simulink model "AgrivoltaicPlatformBasic5_28"  (R2023b)
settings: Solver=VariableStepAuto  StartTime=0.0  StopTime=Tsim  RelTol=1e-3
undefined symbols (not defined in the file or in its folder): Boostparams, Buckparams, Ion, Lithium, PVparams
libraries: fl_lib x18, ee_lib x8, spsSeriesRLCBranchLib x6, nesl_utility x6, spsDiodeLib x2, spsMosfetLib x2, spsPVArrayLib x2, spsVoltageMeasurementLib x2, spsBatteryLib x1, spsCurrentVoltageSimscapeInterfaceLib x1, spsGroundLib x1, sps_lib x1
settings Model: Creator=akoer  LastModifiedBy=akoer
settings DebuggingCC: SignalInfNanChecking=error

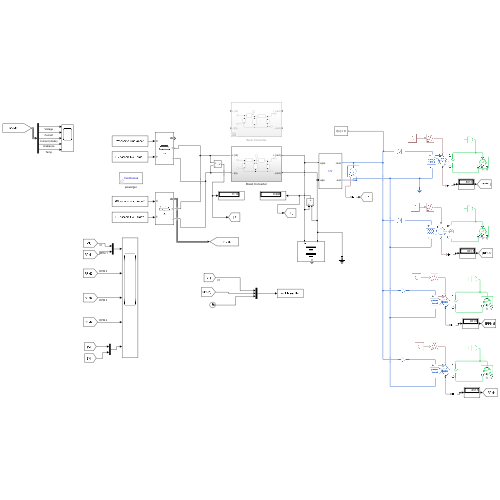
[thumbnail: Simulink's stored preview of the top-level diagram]
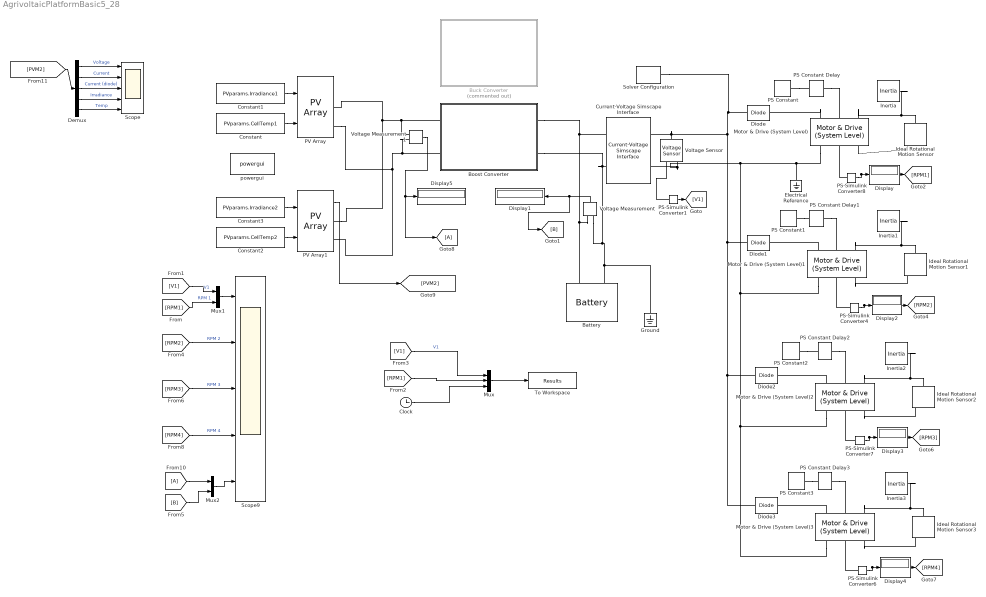
== system AgrivoltaicPlatformBasic5_28 ==
  Battery : spsBatteryLib/Battery  BatType=Lithium-Ion  ShowTempParam=off  ThermalPreset=no  ShowAgeParam=off  NomV=7.2  NomQ=20  SOC=20  Batt_Tr=30  PresetModel=on  MaxQ=20  MinV=5.4  FullV=8.3807  Dis_rate=8.6957  R=0.0036  Normal_OP=18.087  expZone="[7.7788     0.98261]"  current=[6.5 13 32.5]  Units=Time  Tci=20  NomT=20  T2=-30  MaxQ2=4.8  FullV2=7.1  Normal_OP2=5.655  expZone2="[6.58           1]"  Rca=0.6  ti=2000  Dp=0  Neq0=0  Tsim=1e6  Ta1=25  Qeol=5.4*0.9  Reol=0.013333*1.2  Char_age=[2.3478, 3]  Dis_age=[2.3478, 10]  N1=1500  N2=10500  N3=1000  N4=1400  Ta2=45  N5=950
  Boost Converter : Subsystem
  Buck Converter : Subsystem  Commented=on
  Clock : Clock
  Constant : Constant  Value=PVparams.CellTemp1
  Constant1 : Constant  Value=PVparams.Irradiance1
  Constant2 : Constant  Value=PVparams.CellTemp2
  Constant3 : Constant  Value=PVparams.Irradiance2
  Current-Voltage Simscape Interface : spsCurrentVoltageSimscapeInterfaceLib/Current-Voltage Simscape Interface  DFT=on  FMode=Low pass filter (continuous)  T=1e-6  Ts=50e-6  i0=0  v0=0  Sd=Specialized Power Systems side  Measurements=off
      settings: LibrarySourceBlock=|
      | sps_lib/Utilities/Current-Voltage
      | Simscape Interface
  Demux : Demux  Outputs=5
  Diode{,1..3} (4 alike) : ee_lib/Semiconductors & Converters/Diode  ModelType=ee.enum.diode.modelType.pwl  TableType=ee.enum.diode.tableType.IfMat  IfMat=[.07, .12, .19, 1.75, 4.24, 7.32, 11.2; .16, .3, .72, 2.14, 5.02, 8.35, 13.12] A  VfMat=[.9, 1.15, 1.25, 1.5, 1.75, 2.17, 2.6, 2.85; .58, .68, .75, 1.1, 1.38, 1.77, 2.27, 2.7] V  TjVec=[25, 125] degC  VfVec=[.5, .7, .9, 1.3, 1.7, 2.1, 2.5] V  IfVec=[.1, .2, .5, 1, 2, 4, 7, 10] A  Vf=0.6 V  Ron=0.3 Ohm  Goff=1e-8 S  prmExp=ee.enum.diode.expParam.useTwo  I12=[.0137, .545] A  V12=[.6, .7] V  RS=0 Ohm  Tmeas=25 degC  IS=1e-12 A  ec=1  I1=0.0137 A  V1=0.6 V  N_series=1  N_parallel=1  ZenerEnable=false  Rz=0.3 Ohm  BV=inf V  C_param=ee.enum.diode.capParam.fixed  CJ=0 pF  CJ0=5 pF  Vvec=[.1, 10, 100] V  Cvec=[3.5, 1, .4] pF  VJ=1 V  Mgrad=0.5  FC=0.5  Q_param=ee.enum.diode.recoveryParam.off  iRM=-7.15 A  iF=4 A  didt=-750 A/us  trr_factor=3  trr=115 ns  Qrr=150 nA*s  Vr=-600 V  Ls=150 nH  Erec=0.03 J  TT=50 ns  tau=100 ns  T_param=ee.enum.diode.temperatureParam.off  Tdevice=25 degC  I1_T2=0.245 A  V1_T2=0.5 V  IS_T2=1.25e-7 A  Tmeas2=125 degC  XTI_param=ee.enum.diode.xtiParam.pn  XTI=3  EG_param=ee.enum.diode.egapParam.material_si  EG=1.11 eV  dBVdT=0 V/K  enable_faults=simscape.enum.onoff.off  fault_action=simscape.enum.assert.action.none  fault_types=ee.enum.diode.faults.open  tau_fault=1e-3 s  IfMat_faulted=[.07, .12, .19, 1.75, 4.24, 7.32, 11.2; .16, .3, .72, 2.14, 4.02, 6.35, 9.12] A  VfMat_faulted=[.9, 1.15, 1.25, 1.5, 1.75, 2.17, 2.6, 2.85; .58, .68, .75, 1.1, 1.38, 1.77, 2.27, 2.7] V  VfVec_faulted=[.5, .7, .9, 1.3, 1.7, 2.1, 2.5] V  IfVec_faulted=[.1, .2, .5, 1, 2, 4, 7, 10] A  Ropen_faulted=1000 Ohm  Gshort_faulted=1000 1/Ohm  Vf_faulted=0.6 V  Ron_faulted=0.3 Ohm  Goff_faulted=1e-8 S  I12_faulted=[.0137, .545] A  V12_faulted=[.6, .7] V  IS_faulted=1e-12 A  ec_faulted=1  I1_faulted=0.0137 A  V1_faulted=0.6 V  RS_faulted=0 Ohm  Rz_faulted=0.3 Ohm  BV_faulted=inf V  Cscale_faulted=100  fault_trigger=ee.enum.faults.faultTrigger.temporal  t_fault=inf s  max_permissible_voltage=inf V  n_fail_on_voltage=1  max_permissible_current=inf A  t_fail_on_current=1 s  max_permissible_dVdt=inf V/s  enable_fault_input=simscape.enum.onoff.off  i_specify=off  i_priority=None  i=0 A  i_nominal_specify=off  i_nominal_unit=A  i_nominal_value=1  v_specify=off  v_priority=None  v=0 V  v_nominal_specify=off  v_nominal_unit=V  v_nominal_value=1  v_capacitor_specify=off  v_capacitor_priority=None  v_capacitor=0 V  v_capacitor_nominal_specify=off  v_capacitor_nominal_unit=V  v_capacitor_nominal_value=1  faulted_specify=off  faulted_priority=None  faulted=0  faulted_nominal_specify=off  faulted_nominal_unit=1  faulted_nominal_value=1  i_diode_specify=off  i_diode_priority=None  i_diode=0 A  i_diode_nominal_specify=off  i_diode_nominal_unit=A  i_diode_nominal_value=1  v_diode_specify=off  v_diode_priority=None  v_diode=0 V  v_diode_nominal_specify=off  v_diode_nominal_unit=V  v_diode_nominal_value=1  i_capacitor_specify=off  i_capacitor_priority=None  i_capacitor=0 A  i_capacitor_nominal_specify=off  i_capacitor_nominal_unit=A  i_capacitor_nominal_value=1  power_dissipated_specify=off  power_dissipated_priority=None  power_dissipated=0 W  power_dissipated_nominal_specify=off  power_dissipated_nominal_unit=W  power_dissipated_nominal_value=1  fidelity_level=ee.enum.diode.fidelity.includeChargeDyn  rec_loss_model=ee.enum.diode.reverseRecoveryModel.fixed  ErecVal=0 J  scaleWithIandV=true  ErecMat=zeros(2, 3) J  TjrecVec=[298.15, 398.15] K  IfrecVec=[.1, 1, 10] A  IrecVal=10 A  VrecVal=10 V  tFilter=1 / 1000 / 100 s  max_permissible_temperature=inf K  t_fail_on_temperature=1 s  thermal_network_parameterization=ee.enum.thermalNetworkTopology.junctionCase  Rth=[0, 10] K/W  Rth_Cauer=[1, 3, 10] K/W  Rth_Foster=[4, 6] K/W  thermal_mass_parameterization=ee.enum.thermalNetwork.timeconstant  thermal_mass=[0, 1] J/K  thermal_mass_Cauer=[.1, .3, 1] J/K  thermal_mass_Foster=[1.5, 3] J/K  thermal_time_constant=[0, 10] s  thermal_time_constant_Cauer=[1, 3, 10] s  thermal_time_constant_Foster=[6, 18] s  thermal_mass_initial_temperatures=[25, 25] degC  thermal_mass_initial_temperatures_Cauer=[25, 25, 25] degC  junction_thermal_mass=0.01 J/K  Tvec_initial_Foster=[25, 25, 25, 25] degC  no_thermal_network=0  junction_temperature_specify=off  junction_temperature_priority=None  junction_temperature=25 degC  junction_temperature_nominal_specify=off  junction_temperature_nominal_unit=degC  junction_temperature_nominal_value=1
  Display{,1..5} (6 alike) : Display
  Electrical Reference : fl_lib/Electrical/Electrical Elements/Electrical Reference
  From10 : From
  Goto8 : Goto
  Ground : spsGroundLib/Ground  LConnTagsString=a
  Ideal Rotational Motion Sensor{,1..3} (4 alike) : fl_lib/Mechanical/Mechanical Sensors/Ideal Rotational Motion Sensor  reference=foundation.enum.MeasurementReference.difference  acceleration_port=false  velocity_port=true  position_port=true  wrap_angle=false  offset=0 rad
  Inertia{,1..3} (4 alike) : fl_lib/Mechanical/Rotational Elements/Inertia  inertia=params.Inertia kg*m^2  num_ports=foundation.enum.numPorts2.one  w_specify=off  w_priority=High  w=0 rad/s  w_nominal_specify=off  w_nominal_unit=rad/s  w_nominal_value=1  t_specify=off  t_priority=None  t=0 N*m  t_nominal_specify=off  t_nominal_unit=N*m  t_nominal_value=1
  Motor & Drive (System Level){,1..3} (4 alike) : ee_lib/Electromechanical/Motor & Drive (System Level)  torque_speed_param=ee.enum.electromech.envelope.tabulated2D  overtorque_param=ee.enum.electromech.overtorque.no  T_t=[.09, .08, .07, 0] N*m  T_t_intermittent=[.36, .32, .28, 0] N*m  T_t_2D=[.09, .09, .09; .08, .08, .08; .07, .07, .07; 0, 0, 0] N*m  T_t_intermittent_2D=[.36, .36, .36; .32, .32, .32; .28, .28, .28; 0, 0, 0] N*m  w_t=[0, 3750, 7500, 8000] rpm  vdc_t=[6, 12, 24] V  torque_max=0.1 N*m  power_max=30 W  torque_max_intermittent=0.4 N*m  power_max_intermittent=120 W  time_overtorque=30 s  time_recover=60 s  Tc=0.02 s  EnableSwitch=false  losses_param=1  eff=100  w_eff=3750 rpm  T_eff=0.08 N*m  Piron=0 W  Pbase=0 W  w_eff_vec=[-8000, -4000, 0, 4000, 8000] rpm  T_eff_vec=[0, .03, .06, .09] N*m  v_eff_vec=[100, 250, 400] V  losses_mat=[1.49, 1.67, 2.21, 3.1; .42, .69, 1.14, 2.03; .06, .24, .78, 1.68; .42, .69, 1.14, 2.03; 1.49, 1.67, 2.21, 3.1] W  efficiency_mat=[95, 95, 95, 95; 95, 95, 95, 95; 95, 95, 95, 95; 95, 95, 95, 95; 95, 95, 95, 95]  losses_mat_3D=ones(5, 4, 3) W  efficiency_mat_3D=95 * ones(5, 4, 3)  Res=0 Ohm  enable_fault=simscape.enum.onoff.off  fault_condition=1  fault_threshold=0.5  J=5e-5 kg*m^2  lam=1e-5 N*m*s/rad  speed0=0 rpm  faulted_specify=off  faulted_priority=None  faulted=0  faulted_nominal_specify=off  faulted_nominal_unit=1  faulted_nominal_value=1  isSwitchedOff_specify=off  isSwitchedOff_priority=None  isSwitchedOff=0  isSwitchedOff_nominal_specify=off  isSwitchedOff_nominal_unit=1  isSwitchedOff_nominal_value=1  torqueLimitContinuous_specify=off  torqueLimitContinuous_priority=None  torqueLimitContinuous=0 N*m  torqueLimitContinuous_nominal_specify=off  torqueLimitContinuous_nominal_unit=N*m  torqueLimitContinuous_nominal_value=1  alpha=3.93e-3 1/K  Tmeas=25 degC  Tmeas2=125 degC  losses_mat_T2=[1.49, 1.74, 2.49, 3.74; .42, .67, 1.42, 2.67; .06, .31, 1.06, 2.31; .42, .67, 1.42, 2.67; 1.49, 1.74, 2.49, 3.74] W  efficiency_mat_T2=[95, 95, 95, 95; 95, 95, 95, 95; 95, 95, 95, 95; 95, 95, 95, 95; 95, 95, 95, 95]  losses_mat_3D_T2=ones(5, 4, 3) W  efficiency_mat_3D_T2=95 * ones(5, 4, 3)  thermal_mass=100 J/K  initial_temperature=25 degC
  Mux : Mux  Inputs=3
  Mux1 : Mux  Inputs=2
  Mux2 : Mux  Inputs=2
  PS Constant : fl_lib/Physical Signals/Sources/PS Constant  constant=params.Torque1 N*m
  PS Constant Delay{,1..3} (4 alike) : fl_lib/Physical Signals/Delays/PS Constant Delay  InputHistory=0.0 N*m  DelayTime=1.0 s
      settings: InternalSimscapePortConfiguration="{\"Bottom\":[],\"Left\":[{\"id\":\"U\",\"label\":\"U\",\"type\":\"input\"}],\"Right\":[{\"id\":\"Y\",\"label\":\"Y\",\"type\":\"output\"}],\"Top\":[]}"
  PS Constant1 : fl_lib/Physical Signals/Sources/PS Constant  constant=params.Torque2 N*m
  PS Constant2 : fl_lib/Physical Signals/Sources/PS Constant  constant=params.Torque3 N*m
  PS Constant3 : fl_lib/Physical Signals/Sources/PS Constant  constant=params.Torque4 N*m
  PS-Simulink Converter{1,4,6..8} (5 alike) : nesl_utility/PS-Simulink Converter  PhysicalDomain=network_engine_domain  SubClassName=ps_output  LeftPortType=input  RightPortType=output  PseudoPeriodic=off  Frequencies=[]  VectorFormat=inherit  Unit=inherit  AffineConversion=off
  PV Array : spsPVArrayLib/PV Array  Npar=PVparams.Parallel1  Nser=PVparams.Series1  PlotType=array @ 1000 W/m2 & specified temperatures  S_vec="[ 1000  500  100 ]"  Temp_C_vec="[ 45 25  ]"  ModuleName=American Solar Wholesale ASW-185M  PlotWhenSelected=off  Pm=185.13  Ncell=72  Voc=44.6  Isc=5.37  Vm=37.4  Im=4.95  beta_Voc_pc=-0.38595  alpha_Isc_pc=0.043594  beta_Voc=-0.17213  alpha_Isc=0.002341  IL=5.3768  I0=4.1873e-10  nI=1.0375  Rsh=226.7768  Rs=0.28792  RobustModel=off  RobustCellTemperature=313.3991  BAL=on  Tc=1e-6  Tfilter=5e-5
  PV Array1 : spsPVArrayLib/PV Array  Npar=PVparams.Parallel2  Nser=PVparams.Series2  PlotType=array @ 1000 W/m2 & specified temperatures  S_vec="[ 1000  500  100 ]"  Temp_C_vec="[ 45 25  ]"  ModuleName=American Solar Wholesale ASW-185M  PlotWhenSelected=off  Pm=185.13  Ncell=72  Voc=44.6  Isc=5.37  Vm=37.4  Im=4.95  beta_Voc_pc=-0.38595  alpha_Isc_pc=0.043594  beta_Voc=-0.17213  alpha_Isc=0.002341  IL=5.3768  I0=4.1873e-10  nI=1.0375  Rsh=226.7768  Rs=0.28792  RobustModel=off  RobustCellTemperature=313.3991  BAL=on  Tc=1e-6  Tfilter=5e-5
  Scope : Scope  NumInputPorts=5
  Scope9 : Scope  NumInputPorts=5
  Solver Configuration : nesl_utility/Solver Configuration  PhysicalDomain=network_engine_domain  SubClassName=solver  LeftPortType=input  RightPortType=generic  Tones=[]  Harmonics=[]  SimulateNoise=off  Profile=off  UseLocalSampling=off  EnableSwitchedLinearOptims=on  FrequencyDomain=off  UseCCode=off  RelTol=0.001  AbsTol=0.001  MinStep=1e-09  ToWorkspace=off  RevertToSquareIcSolve=off  NumHomotopyIterations=100  PhasorMode=off  PhasorModeNumHarmonics=1  ConsistencySolver=NEWTON_XTOL_AFTER_FTOL  IndexReductionMethod=DerivativeReplacement  DoDC=off  ResidualTolerance=1e-09  ConsistencyTolSource=GLOBAL  ConsistencyAbsTol=0.001  ConsistencyRelTol=0.001  ConsistencyTolFactor=0.001  UseLocalSolver=off  LocalSolverChoice=NE_BACKWARD_EULER_ADVANCER  ResolveIndetEquations=on  FunctionEvalNumThread=1  LocalSolverSampleTime=0.001  DoFixedCost=off  MaxNonlinIter=3  MaxModeIter=2  ComputeImpulses=off  ImpulseIterations=2  LinearAlgebra=auto  LinearAlgebraNumThread=0  EquationFormulation=NE_TIME_EF  DelaysMemoryBudget=1024  AutomaticFiltering=on  FilteringTimeConstant=0.001  PartitionStorageMethod=AS_NEEDED  PartitionMemoryBudget=1024  PartitionMethod=ROBUST  MultibodyUseLocalSolver=off  MultibodyLocalSolverChoice=ODE1  MultibodyLocalSolverSampleTime=0.001
  To Workspace : ToWorkspace  VariableName=Results  SampleTime=-1
  Voltage Measurement : spsVoltageMeasurementLib/Voltage Measurement  PhasorSimulation=off  OutputType=Complex  PSBequivalent=0
  Voltage Measurement1 : spsVoltageMeasurementLib/Voltage Measurement  PhasorSimulation=off  OutputType=Complex  PSBequivalent=0
  Voltage Sensor : fl_lib/Electrical/Electrical Sensors/Voltage Sensor
  powergui : sps_lib/powergui  Priority=1  SimulationMode=Continuous  SampleTime=50e-4  frequency=60  Iterations=50  frequencyindice=0  Pbase=100e6  ErrMax=1e-4  UnitsV=kV  UnitsW=MW  buscounter=0  FunctionMessages=off  echomessages=off  EnableUseOfTLC=off  CurrentSourceSwitches=off  DisableSnubberDevices=off  DisableRonSwitches=off  DisableVfSwitches=off  DisplayEquations=off  AutomaticDiscreteSolvers=off  SolverType=Tustin/Backward Euler (TBE)  Interpol=off  ExternalGateDelay=off  methode=off  Ts=100  x0status=blocks  SPID=on  SwTol=0  HookPort=off  NonlinearTolerance=1e-4  nMaxIteration=100  ContinueOnMaxIteration=off  RestoreLinks=warning  ResistiveCurrentMeasurement=off  Frange=[0:2:500]  Ylog=off  Xlog=on  ShowGrid=off  save=off  variable=ZData  structure=0  ZoomFFT=off  StartTime=0.0  cycles=1  DisplayStyle=1  fundamental=60  FreqAxis=off  MaxFrequency=1000  frequencyindicesteady=1  RmsSteady=1  display=off
  wires:
  Constant/1 -> PV Array/2
  Constant1/1 -> PV Array/1
  Voltage Measurement/1 -> [B], Display1/1
  Constant3/1 -> PV Array1/1
  Constant2/1 -> PV Array1/2
  PS-Simulink Converter1/1 -> [V1]
  [V1] -> Mux/1  "V1"
  Mux/1 -> To Workspace/1
  [RPM1] -> Mux/2
  [RPM1] -> Mux1/2  "RPM 1"
  PS-Simulink Converter8/1 -> [RPM1], Display/1
  Clock/1 -> Mux/3
  Mux1/1 -> Scope9/1
  [V1] -> Mux1/1  "V1"
  [RPM2] -> Scope9/2  "RPM 2"
  PS-Simulink Converter4/1 -> [RPM2], Display2/1
  PS-Simulink Converter6/1 -> [RPM4], Display4/1
  PS-Simulink Converter7/1 -> [RPM3], Display3/1
  [RPM4] -> Scope9/4  "RPM 4"
  Voltage Measurement1/1 -> Goto8/1, Display5/1
  PV Array1/1 -> [PVM2]
  [RPM3] -> Scope9/3  "RPM 3"
  [PVM2] -> Demux/1
  Demux/1 -> Scope/1  "Voltage"
  Demux/2 -> Scope/2  "Current"
  Demux/3 -> Scope/3  "Current (diode)"
  Demux/4 -> Scope/4  "Irradiance"
  Demux/5 -> Scope/5  "Temp"
  From10/1 -> Mux2/1
  [B] -> Mux2/2
  Mux2/1 -> Scope9/5
  connections:
  Motor & Drive (System Level)/LConn1 -- Diode/RConn1
  Motor & Drive (System Level)/RConn3 -- Ideal Rotational Motion Sensor/RConn1
  Inertia/LConn1 -- Motor & Drive (System Level)/LConn3 -- Ideal Rotational Motion Sensor/LConn1
  PS-Simulink Converter1/LConn1 -- Voltage Sensor/RConn1
  Current-Voltage Simscape Interface/RConn1 -- Diode3/LConn1 -- Diode2/LConn1 -- Diode1/LConn1 -- Solver Configuration/RConn1 -- Diode/LConn1 -- Voltage Sensor/LConn1
  PS Constant/RConn1 -- PS Constant Delay/LConn1
  PS Constant Delay/RConn1 -- Motor & Drive (System Level)/LConn2
  PS-Simulink Converter8/LConn1 -- Motor & Drive (System Level)/RConn2
  Ideal Rotational Motion Sensor1/LConn1 -- Motor & Drive (System Level)1/LConn3 -- Inertia1/LConn1
  Motor & Drive (System Level)1/LConn1 -- Diode1/RConn1
  PS-Simulink Converter4/LConn1 -- Motor & Drive (System Level)1/RConn2
  Motor & Drive (System Level)1/RConn3 -- Ideal Rotational Motion Sensor1/RConn1
  PS Constant Delay1/RConn1 -- Motor & Drive (System Level)1/LConn2
  PS Constant1/RConn1 -- PS Constant Delay1/LConn1
  PV Array1/RConn1 -- Boost Converter/LConn1 -- Voltage Measurement1/LConn1 -- PV Array/RConn1
  Voltage Measurement/LConn1 -- Boost Converter/RConn1 -- Current-Voltage Simscape Interface/LConn1 -- Battery/LConn1
  Current-Voltage Simscape Interface/LConn2 -- Boost Converter/RConn2 -- Ground/LConn1 -- Battery/LConn2 -- Voltage Measurement/LConn2
  Voltage Measurement1/LConn2 -- Boost Converter/LConn2 -- PV Array1/RConn2 -- PV Array/RConn2
  Motor & Drive (System Level)3/LConn1 -- Diode3/RConn1
  Motor & Drive (System Level)2/LConn1 -- Diode2/RConn1
  Ideal Rotational Motion Sensor2/LConn1 -- Motor & Drive (System Level)2/LConn3 -- Inertia2/LConn1
  Ideal Rotational Motion Sensor3/LConn1 -- Motor & Drive (System Level)3/LConn3 -- Inertia3/LConn1
  PS-Simulink Converter7/LConn1 -- Motor & Drive (System Level)2/RConn2
  PS-Simulink Converter6/LConn1 -- Motor & Drive (System Level)3/RConn2
  PS Constant3/RConn1 -- PS Constant Delay3/LConn1
  PS Constant Delay2/RConn1 -- Motor & Drive (System Level)2/LConn2
  PS Constant2/RConn1 -- PS Constant Delay2/LConn1
  PS Constant Delay3/RConn1 -- Motor & Drive (System Level)3/LConn2
  Motor & Drive (System Level)2/RConn3 -- Ideal Rotational Motion Sensor2/RConn1
  Motor & Drive (System Level)3/RConn3 -- Ideal Rotational Motion Sensor3/RConn1
  Voltage Sensor/RConn2 -- Motor & Drive (System Level)/RConn1 -- Electrical Reference/LConn1 -- Motor & Drive (System Level)3/RConn1 -- Motor & Drive (System Level)2/RConn1 -- Motor & Drive (System Level)1/RConn1 -- Current-Voltage Simscape Interface/RConn2

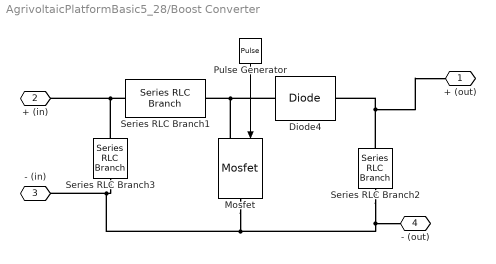
== system AgrivoltaicPlatformBasic5_28/Boost Converter ==
  Diode4 : spsDiodeLib/Diode  Ron=0.001  Lon=0  Vf=0.8  IC=0  UseSnubber=0  Rs=500  Cs=250e-9  Measurements=off
  Mosfet : spsMosfetLib/Mosfet  Ron=0.1  Lon=0  Rd=0.01  Vfd=0  IC=0  Rs=1e5  Cs=inf  Measurements=off
  Pulse Generator : DiscretePulseGenerator  PulseType=Time based  Period=Boostparams.Tau  PulseWidth=Boostparams.MosfetPWM
  Series RLC Branch1 : spsSeriesRLCBranchLib/Series RLC Branch  LConnTagsString=__new0  RConnTagsString=__new0  BranchType=L  Resistance=1  Inductance=Boostparams.L  SetiL0=off  InitialCurrent=0  Capacitance=1e-6  Setx0=off  InitialVoltage=0  Measurements=None
  Series RLC Branch2 : spsSeriesRLCBranchLib/Series RLC Branch  LConnTagsString=__new0  RConnTagsString=__new0  BranchType=C  Resistance=1  Inductance=1e-3  SetiL0=off  InitialCurrent=0  Capacitance=Boostparams.Cout  Setx0=off  InitialVoltage=0  Measurements=None
  Series RLC Branch3 : spsSeriesRLCBranchLib/Series RLC Branch  LConnTagsString=__new0  RConnTagsString=__new0  BranchType=C  Resistance=1  Inductance=1e-3  SetiL0=off  InitialCurrent=0  Capacitance=Boostparams.Cin  Setx0=on  InitialVoltage=.1  Measurements=None
  + (out) : PMIOPort  Side=Right
  + (in) : PMIOPort  Port=2  Side=Left
  - (in) : PMIOPort  Port=3  Side=Left
  - (out) : PMIOPort  Port=4  Side=Right
  wires:
  Pulse Generator/1 -> Mosfet/1
  connections:
  Series RLC Branch2/LConn1 -- + (out)/RConn1 -- Diode4/RConn1
  Series RLC Branch3/LConn1 -- + (in)/RConn1 -- Series RLC Branch1/LConn1
  Diode4/LConn1 -- Mosfet/LConn1 -- Series RLC Branch1/RConn1
  Series RLC Branch2/RConn1 -- - (in)/RConn1 -- Series RLC Branch3/RConn1 -- Mosfet/RConn1 -- - (out)/RConn1

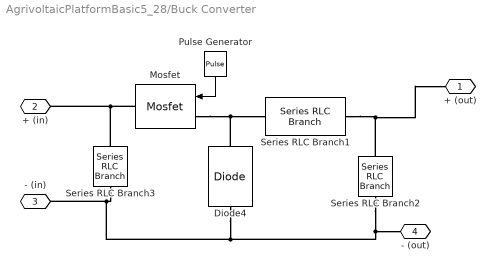
== system AgrivoltaicPlatformBasic5_28/Buck Converter ==
  Diode4 : spsDiodeLib/Diode  Ron=0.001  Lon=0  Vf=0.8  IC=0  UseSnubber=0  Rs=500  Cs=250e-9  Measurements=off
  Mosfet : spsMosfetLib/Mosfet  Ron=0.1  Lon=0  Rd=0.01  Vfd=0  IC=0  Rs=1e5  Cs=inf  Measurements=off
  Pulse Generator : DiscretePulseGenerator  PulseType=Time based  Period=10  PulseWidth=Buckparams.MosfetPWM
  Series RLC Branch1 : spsSeriesRLCBranchLib/Series RLC Branch  LConnTagsString=__new0  RConnTagsString=__new0  BranchType=L  Resistance=1  Inductance=Buckparams.L  SetiL0=off  InitialCurrent=0  Capacitance=1e-6  Setx0=off  InitialVoltage=0  Measurements=None
  Series RLC Branch2 : spsSeriesRLCBranchLib/Series RLC Branch  LConnTagsString=__new0  RConnTagsString=__new0  BranchType=C  Resistance=1  Inductance=1e-3  SetiL0=off  InitialCurrent=0  Capacitance=Buckparams.Cout  Setx0=off  InitialVoltage=0  Measurements=None
  Series RLC Branch3 : spsSeriesRLCBranchLib/Series RLC Branch  LConnTagsString=__new0  RConnTagsString=__new0  BranchType=C  Resistance=1  Inductance=1e-3  SetiL0=off  InitialCurrent=0  Capacitance=Buckparams.Cin  Setx0=on  InitialVoltage=1  Measurements=None
  + (out) : PMIOPort  Side=Right
  + (in) : PMIOPort  Port=2  Side=Left
  - (in) : PMIOPort  Port=3  Side=Left
  - (out) : PMIOPort  Port=4  Side=Right
  wires:
  Pulse Generator/1 -> Mosfet/1
  connections:
  Series RLC Branch2/LConn1 -- Series RLC Branch1/RConn1 -- + (out)/RConn1
  Series RLC Branch3/LConn1 -- Mosfet/RConn1 -- + (in)/RConn1
  - (in)/RConn1 -- Diode4/LConn1 -- Series RLC Branch2/RConn1 -- - (out)/RConn1 -- Series RLC Branch3/RConn1
  Mosfet/LConn1 -- Diode4/RConn1 -- Series RLC Branch1/LConn1
